simulink model "FinalV2"  (R2018b)
settings: Solver=FixedStepAuto  StartTime=0.0  StopTime=1  RelTol=1e-3
values from neighbouring files (symbols this model uses):
  Kdi = dlqr(Ad,Bd,Q,R)    [finalScript.m]    (also in finalScriptV2.m)
  n = 16.5    [DC_motor_geared_integral_discrete_sysid23.m]    (also in DC_motor_geared_lqr_discrete_sysid23.m; finalScript.m; finalScriptV2.m)
  Tsc = 1/20000    (= 5e-05)    [DC_motor_geared_integral_discrete_sysid23.m]    (also in DC_motor_geared_lqr_discrete_sysid23.m = 1e-05; finalScript.m; finalScriptV2.m = 0.001)
undefined symbols (not defined in the file or in its folder): DiscIntNeverNeededParam
libraries: dspswit3 x29, mbedblockslib x19, simulink x10, dspsigops x5, powerlib_meascontrol x4, dspstat3 x2, peGeneralControl x1
(part 1 of 2)
settings Model: Creator=Roberto  LastModifiedBy=Cas
settings SolverCC: AutoInsertRateTranBlk=on
settings OptimizationCC: DefaultParameterBehavior=Inlined  UseFloatMulNetSlope=on  UseSpecifiedMinMax=on  InlineInvariantSignals=on  PassReuseOutputArgsAs=Individual arguments  ZeroExternalMemoryAtStartup=off  ZeroInternalMemoryAtStartup=off  NoFixptDivByZeroProtection=on  EfficientFloat2IntCast=on  MaxStackSize=64  OptimizeBlockOrder=speed  DifferentSizesBufferReuse=on
settings DebuggingCC: ParameterTunabilityLossMsg=error
settings HardwareCC: ProdBitPerPointer=32  ProdBitPerSizeT=32  ProdBitPerPtrDiffT=32  ProdLargestAtomicInteger=Long  ProdLargestAtomicFloat=Double  ProdWordSize=32  ProdLongLongMode=on  ProdHWDeviceType=ARM Compatible->ARM Cortex
settings ModelReferenceCC: ModelReferenceMinAlgLoopOccurrences=on
settings SFSimCC: MATLABDynamicMemAlloc=off
settings RTWCC: SystemTargetFile=ert.tlc  HardwareBoard=STM32F746G-Discovery  TemplateMakefile=ert_default_tmf  GenerateReport=on  Toolchain=GNU Tools for ARM Embedded Processors  BuildConfiguration=Faster Runs  IncludeHyperlinkInReport=on  LaunchReport=on  GenerateTraceInfo=on  GenerateTraceReport=on  GenerateTraceReportSl=on  GenerateTraceReportSf=on  GenerateTraceReportEml=on
settings CodeAppCC: ForceParamTrailComments=on  IgnoreCustomStorageClasses=off  OperatorAnnotations=on  SimulinkDataObjDesc=on  SFDataObjDesc=on  InsertBlockDesc=on
settings ERTTargetCC: CombineSignalStateStructs=on  SuppressErrorStatus=on  SupportNonFinite=off

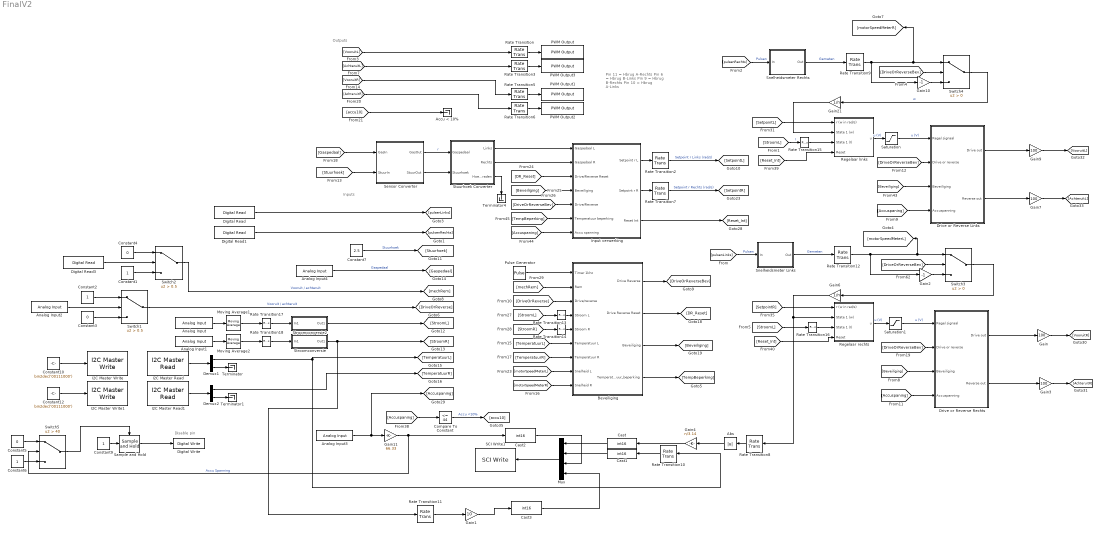
== system FinalV2 ==
  note: Disable pin
  note: Pin 11 = Hbrug A-Rechts
      | Pin 6   = Hbrug B-Links
      | Pin 9   = Hbrug B-Rechts
      | Pin 10 = Hbrug A-Links
  note: Inputs
  note: Outputs
  Abs : Abs
  Accu < 10% : Terminator
  Analog Input : mbedblockslib/Analog Input  Pin=A3  ReadResultsOnly=off  ConversionTriggerSource=Software  ExternalTriggerType=uint32( 0 )  OutputDataType=double  EnableConversionCompleteNotify=off  EnableOuputStatus=off  SampleTime=1/10000
      settings: SourceProductName=Simulink Coder Support Package for BBC microbit Board  SourceProductBaseCode=MICROBIT
  Analog Input1 : mbedblockslib/Analog Input  Pin=A2  ReadResultsOnly=off  ConversionTriggerSource=Software  ExternalTriggerType=uint32( 0 )  OutputDataType=double  EnableConversionCompleteNotify=off  EnableOuputStatus=off  SampleTime=1/10000
      settings: SourceProductName=Simulink Coder Support Package for BBC microbit Board  SourceProductBaseCode=MICROBIT
  Analog Input2 : mbedblockslib/Analog Input  Pin=A0  ReadResultsOnly=off  ConversionTriggerSource=Software  ExternalTriggerType=uint32( 0 )  OutputDataType=double  EnableConversionCompleteNotify=off  EnableOuputStatus=off  SampleTime=Tsc
      settings: SourceProductName=Simulink Coder Support Package for BBC microbit Board  SourceProductBaseCode=MICROBIT
  Analog Input3 : mbedblockslib/Analog Input  Pin=A1  ReadResultsOnly=off  ConversionTriggerSource=Software  ExternalTriggerType=uint32( 0 )  OutputDataType=double  EnableConversionCompleteNotify=off  EnableOuputStatus=off  SampleTime=1/20
      settings: SourceProductName=Simulink Coder Support Package for BBC microbit Board  SourceProductBaseCode=MICROBIT
  Analog Input4 : mbedblockslib/Analog Input  Pin=A4  ReadResultsOnly=off  ConversionTriggerSource=Software  ExternalTriggerType=uint32( 0 )  OutputDataType=double  EnableConversionCompleteNotify=off  EnableOuputStatus=off  SampleTime=Tsc
      settings: SourceProductName=Simulink Coder Support Package for BBC microbit Board  SourceProductBaseCode=MICROBIT
  Beveiliging : Subsystem
  Cast{,1..3} (4 alike) : DataTypeConversion  OutDataTypeStr=int16
  Compare To Constant : simulink/Logic and Bit Operations/Compare To Constant  relop=<=  const=44  OutDataTypeStr=boolean
  Constant1 : Constant  OutDataTypeStr=boolean  SampleTime=Tsc
  Constant10 : Constant  Value=bin2dec('00111000')  OutDataTypeStr=uint8  SampleTime=20
  Constant12 : Constant  Value=bin2dec('00111000')  OutDataTypeStr=uint8  SampleTime=20
  Constant2 : Constant  OutDataTypeStr=boolean  SampleTime=Tsc
  Constant3 : Constant  Value=0  OutDataTypeStr=boolean  SampleTime=Tsc
  Constant4 : Constant  Value=0  OutDataTypeStr=boolean  SampleTime=Tsc
  Constant5 : Constant  Value=0  OutDataTypeStr=boolean  SampleTime=1/20
  Constant6 : Constant  OutDataTypeStr=boolean  SampleTime=1/20
  Constant7 : Constant  Value=2.5  SampleTime=Tsc
  Constant9 : Constant  OutDataTypeStr=boolean  SampleTime=1/20
  Demux1 : Demux  Outputs=2
  Demux2 : Demux  Outputs=2
  Digital Read : mbedblockslib/Digital Read  Pin=4  Direction=input  SampleTime=1/200000
      settings: SourceProductName=Simulink Coder Support Package for BBC microbit Board  SourceProductBaseCode=MICROBIT
  Digital Read1 : mbedblockslib/Digital Read  Pin=5  Direction=input  SampleTime=1/200000
      settings: SourceProductName=Simulink Coder Support Package for BBC microbit Board  SourceProductBaseCode=MICROBIT
  Digital Read3 : mbedblockslib/Digital Read  Pin=2  Direction=input  SampleTime=Tsc
      settings: SourceProductName=Simulink Coder Support Package for BBC microbit Board  SourceProductBaseCode=MICROBIT
  Digital Write : mbedblockslib/Digital Write  Pin=7  Direction=output
      settings: SourceProductName=Simulink Coder Support Package for BBC microbit Board  SourceProductBaseCode=MICROBIT
  Drive or Reverse Links : Subsystem
  Drive or Reverse Rechts : Subsystem
  Gain{,3,7,9} (4 alike) : Gain  Gain=100
  Gain1 : Gain  Gain=10
  Gain10 : Gain  Gain=-1
  Gain11 : Gain  Gain=66.33
  Gain2 : Gain  Gain=-1
  Gain21 : Gain  Gain=1/n
  Gain4 : Gain  Gain=n/3.14
  Gain6 : Gain  Gain=1/n
  I2C Master Read : mbedblockslib/I2C Master Read  I2CModule=0  Mode=Master  SlaveAddress=bin2dec('1001001')  SlaveByteOrder=BigEndian  Direction=Receiver  RegisterAddressMode=on  RegisterAddress=uint8(0)  SlaveDataType=uint8  DataLength=2  NoAck=off  RepeatedStart=off  OutputStatus=off  SampleTime=1/1000
      settings: SourceProductName=Simulink Coder Support Package for BBC microbit Board  SourceProductBaseCode=MICROBIT
  I2C Master Read1 : mbedblockslib/I2C Master Read  I2CModule=0  Mode=Master  SlaveAddress=bin2dec('1001000')  SlaveByteOrder=BigEndian  Direction=Receiver  RegisterAddressMode=on  RegisterAddress=uint8(0)  SlaveDataType=uint8  DataLength=2  NoAck=off  RepeatedStart=off  OutputStatus=off  SampleTime=1/1000
      settings: SourceProductName=Simulink Coder Support Package for BBC microbit Board  SourceProductBaseCode=MICROBIT
  I2C Master Write : mbedblockslib/I2C Master Write  I2CModule=0  Mode=Master  SlaveAddress=bin2dec('1001001')  SlaveByteOrder=BigEndian  Direction=Transmitter  RegisterAddressMode=on  RegisterAddress=uint8(1)  SlaveDataType=uint8  DataLength=2  NoAck=off  RepeatedStart=off  OutputStatus=off
      settings: SourceProductName=Simulink Coder Support Package for BBC microbit Board  SourceProductBaseCode=MICROBIT
  I2C Master Write1 : mbedblockslib/I2C Master Write  I2CModule=0  Mode=Master  SlaveAddress=bin2dec('1001000')  SlaveByteOrder=BigEndian  Direction=Transmitter  RegisterAddressMode=on  RegisterAddress=uint8(1)  SlaveDataType=uint8  DataLength=2  NoAck=off  RepeatedStart=off  OutputStatus=off
      settings: SourceProductName=Simulink Coder Support Package for BBC microbit Board  SourceProductBaseCode=MICROBIT
  Input verwerking : Subsystem
  Moving Average1 : dspstat3/Moving Average  Method=Sliding window  ForgettingFactorPort=off  SpecifyWindowLength=on  WindowLength=20  ForgettingFactor=0.9  SimulateUsing=Code generation
  Moving Average2 : dspstat3/Moving Average  Method=Sliding window  ForgettingFactorPort=off  SpecifyWindowLength=on  WindowLength=20  ForgettingFactor=0.9  SimulateUsing=Code generation
  Mux : Mux
  PWM Output : mbedblockslib/PWM Output  Pin=10  EnableInputFrequency=off  InitialFrequency=20e3  InitialDutyCycle=0  NotificationType=None
      settings: SourceProductName=Simulink Coder Support Package for BBC microbit Board  SourceProductBaseCode=MICROBIT
  PWM Output1 : mbedblockslib/PWM Output  Pin=6  EnableInputFrequency=off  InitialFrequency=20e3  InitialDutyCycle=0  NotificationType=None
      settings: SourceProductName=Simulink Coder Support Package for BBC microbit Board  SourceProductBaseCode=MICROBIT
  PWM Output2 : mbedblockslib/PWM Output  Pin=9  EnableInputFrequency=off  InitialFrequency=20e3  InitialDutyCycle=0  NotificationType=None
      settings: SourceProductName=Simulink Coder Support Package for BBC microbit Board  SourceProductBaseCode=MICROBIT
  PWM Output3 : mbedblockslib/PWM Output  Pin=11  EnableInputFrequency=off  InitialFrequency=20e3  InitialDutyCycle=0  NotificationType=None
      settings: SourceProductName=Simulink Coder Support Package for BBC microbit Board  SourceProductBaseCode=MICROBIT
  Pulse Generator : DiscretePulseGenerator  SampleTime=1/1000
  Rate Transition{,3,5..6,8,10..11} (7 alike) : RateTransition  OutPortSampleTime=1/20
  Rate Transition{2,7,9,12,15..18} (8 alike) : RateTransition  OutPortSampleTime=Tsc
  Rate Transition13 : RateTransition  OutPortSampleTime=1/1000
  Rate Transition14 : RateTransition  OutPortSampleTime=1/1000
  Regelaar links : Subsystem
  Regelaar rechts : Subsystem
  SCI Write1 : mbedblockslib/SCI Write  SCIModule=0  Baudrate=uint32(9600)  Parity=None  StopBits=1  HardwareFlowControl=None  ByteOrder=LittleEndian  OutputStatus=off
      settings: SourceProductName=Simulink Coder Support Package for BBC microbit Board  SourceProductBaseCode=MICROBIT
  Sample and Hold : dspsigops/Sample and Hold  trig=Rising edge  initCond=0  latchinput=off
  Saturation : Saturate  UpperLimit=60  LowerLimit=-60  OutDataTypeStr=Inherit: Inherit via back propagation
  Saturation1 : Saturate  UpperLimit=60  LowerLimit=-60
  Sensor Converter : Subsystem
  Snelheidsmeter Links : Subsystem
  Snelheidsmeter Rechts : Subsystem
  Stroomconversie : Subsystem
  Stroomconversie2 : Subsystem
  Stuurhoek Converter : Subsystem
  Switch1 : Switch  Criteria=u2 > Threshold  Threshold=0.5
  Switch2 : Switch  Criteria=u2 > Threshold  Threshold=0.5
  Switch3 : Switch  Criteria=u2 > Threshold
  Switch4 : Switch  Criteria=u2 > Threshold
  Switch5 : Switch  Criteria=u2 > Threshold  Threshold=40
  Terminator : Terminator
  Terminator1 : Terminator
  Terminator4 : Terminator
  wires:
  [pulsenRechts] -> Snelheidsmeter Rechts/1(In)  "Pulsen"
  Beveiliging/1("Drive Reverse ") -> [DriveOrReverseBev]
  [Gaspedaal] -> Sensor Converter/1(GasIn)
  Stuurhoek Converter/1(Links) -> Input verwerking/1(Gaspedaal L)
  Input verwerking/1(Setpoint r L) -> Rate Transition2/1
  [Stuurhoek] -> Sensor Converter/2(StuurIn)
  Input verwerking/3(Reset Int) -> [Reset_Int]
  Sensor Converter/2(StuurOut) -> Stuurhoek Converter/2(Stuurhoek)
  [DriveOrReverse] -> Beveiliging/3(Drive/reverse)
  [TemperatuurL] -> Beveiliging/6(Temperatuur L)
  Beveiliging/3(Beveiliging) -> [Beveiliging]
  Input verwerking/2(Setpoint r R) -> Rate Transition7/1
  Beveiliging/2(Drive Reverse Reset) -> [DR_Reset]
  Stuurhoek Converter/2(Rechts) -> Input verwerking/2(Gaspedaal R)
  [mechRem] -> Beveiliging/2(Rem)
  [DR_Reset] -> Input verwerking/3(Drive/Reverse Reset)
  [Beveiliging] -> Input verwerking/4(Beveiliging)
  Pulse Generator/1 -> Beveiliging/1(Timer 1khz)
  [DriveOrReverseBev] -> Input verwerking/5(Drive/Reverse)
  Rate Transition7/1 -> [SetpointR]  "Setpoint r Rechts (rad/s)"
  Rate Transition2/1 -> [SetpointL]  "Setpoint r Links (rad/s)"
  [TemperatuurR] -> Beveiliging/7(Temperatuur R)
  Snelheidsmeter Links/1(Out) -> Rate Transition12/1  "Gemeten"
  [Reset_Int] -> Regelaar rechts/4(Reset)
  [pulsenLinks] -> Snelheidsmeter Links/1(In)  "Pulsen"
  [SetpointR] -> Regelaar rechts/1(r (w in rad/s))
  [Beveiliging] -> Drive or Reverse Rechts/3(Beveiliging)
  Drive or Reverse Rechts/1(Drive out) -> Gain/1
  [Accuspaning] -> Drive or Reverse Rechts/4(Accuspanning)
  [DriveOrReverseBev] -> Drive or Reverse Rechts/2(Drive or reverse)
  Drive or Reverse Rechts/2(Reverse out) -> Gain3/1
  Regelaar rechts/1(u) -> Saturation1/1  "u (V)"
  [Beveiliging] -> Drive or Reverse Links/3(Beveiliging)
  Drive or Reverse Links/1(Drive out) -> Gain9/1
  [Accuspaning] -> Drive or Reverse Links/4(Accuspanning)
  [DriveOrReverseBev] -> Drive or Reverse Links/2(Drive or reverse)
  Drive or Reverse Links/2(Reverse out) -> Gain7/1
  Regelaar links/1(u) -> Saturation/1  "u (V)"
  Switch1/1 -> [DriveOrReverse]  "Vooruit / achteruit"
  Constant7/1 -> [Stuurhoek]  "Stuurhoek"
  Beveiliging/4(Temperatuur_beperking) -> [TempBeperking]
  [Accuspaning] -> Input verwerking/7(Accu spanning)
  [TempBeperking] -> Input verwerking/6(Temperatuur beperking)
  [DriveOrReverseBev] -> Switch3/2
  Gain2/1 -> Switch3/3
  Gain10/1 -> Switch4/3
  [DriveOrReverseBev] -> Switch4/2
  Saturation/1 -> Drive or Reverse Links/1(Regel signaal)  "u (V)"
  Saturation1/1 -> Drive or Reverse Rechts/1(Regel signaal)  "u (V)"
  Compare To Constant/1 -> [accu10]  "Accu <10%"
  [Accuspaning] -> Compare To Constant/1
  Sensor Converter/1(GasOut) -> Stuurhoek Converter/1("Gaspedaal ")  "r"
  Stuurhoek Converter/3(Hoek in graden) -> Terminator4/1
  Gain/1 -> [VooruitR]
  Gain3/1 -> [AchteruitR]
  Gain7/1 -> [AchteruitL]
  Gain9/1 -> [VooruitL]
  [accu10] -> Accu < 10%/1
  [SetpointL] -> Regelaar links/1(r (w in rad/s))
  Switch4/1 -> Gain21/1  "w"
  [StroomL] -> Rate Transition15/1  "I"
  [Reset_Int] -> Regelaar links/4(Reset)
  Snelheidsmeter Rechts/1(Out) -> Rate Transition9/1  "Gemeten"
  [AchteruitR] -> Rate Transition6/1
  [VooruitR] -> Rate Transition5/1
  Rate Transition3/1 -> PWM Output3/1
  Rate Transition5/1 -> PWM Output1/1
  Rate Transition6/1 -> PWM Output2/1
  Rate Transition/1 -> PWM Output/1
  Digital Read/1 -> [pulsenLinks]
  Analog Input3/1 -> [Accuspaning], Gain11/1
  Analog Input4/1 -> [Gaspedaal]  "Gaspedaal"
  [StroomL] -> Rate Transition16/1
  Constant2/1 -> Switch1/1
  Constant3/1 -> Switch1/3
  Digital Read3/1 -> Switch2/2
  Constant1/1 -> Switch2/3
  Constant4/1 -> Switch2/1
  Switch2/1 -> [mechRem]  "Vooruit / achteruit"
  Analog Input2/1 -> Switch1/2
  I2C Master Read/1 -> Demux1/1
  Constant10/1 -> I2C Master Write/1
  Demux1/2 -> Terminator/1
  Stroomconversie2/1(Out1) -> [StroomL]
  [StroomL] -> Rate Transition13/1
  [StroomR] -> Rate Transition14/1
  Cast1/1 -> Mux/2
  Switch3/1 -> Gain6/1
  Abs/1 -> Gain4/1
  Mux/1 -> SCI Write1/1
  Rate Transition8/1 -> Abs/1
  Rate Transition10/1 -> Cast1/1
  Rate Transition11/1 -> Gain1/1
  Gain1/1 -> Cast3/1
  Gain11/1 -> Switch5/2, Cast2/1  "Accu Spanning"
  Constant6/1 -> Switch5/3
  Constant5/1 -> Switch5/1
  Switch5/1 -> Sample and Hold/Trigger
  Constant9/1 -> Sample and Hold/1
  Sample and Hold/1 -> Digital Write/1
  [VooruitL] -> Rate Transition/1
  [AchteruitL] -> Rate Transition3/1
  Gain4/1 -> Cast/1
  Gain6/1 -> Rate Transition8/1, Regelaar rechts/2(State 1 (w))
  Gain21/1 -> Regelaar links/2(State 1 (w))
  Constant12/1 -> I2C Master Write1/1
  I2C Master Read1/1 -> Demux2/1
  Demux2/2 -> Terminator1/1
  Demux2/1 -> [TemperatuurR]
  Rate Transition9/1 -> Gain10/1, [motorSpeedMeterR], Switch4/1
  Rate Transition12/1 -> Gain2/1, [motorSpeedMeterL], Switch3/1
  [motorSpeedMeterL] -> Beveiliging/8(Snelheid L)
  [motorSpeedMeterR] -> Beveiliging/9(Snelheid R)
  Rate Transition13/1 -> Beveiliging/4(Stroom L)
  Rate Transition14/1 -> Beveiliging/5(Stroom R)
  Rate Transition15/1 -> Regelaar links/3(State 1 (I))
  Rate Transition16/1 -> Regelaar rechts/3(State 1 (I))
  Analog Input/1 -> Moving Average1/1
  Analog Input1/1 -> Moving Average2/1
  Rate Transition17/1 -> Stroomconversie2/1(In1)
  Rate Transition18/1 -> Stroomconversie/1(In1)
  Stroomconversie/1(Out1) -> Rate Transition11/1, [StroomR]
  Moving Average1/1 -> Rate Transition17/1
  Moving Average2/1 -> Rate Transition18/1
  Demux1/1 -> Rate Transition10/1, [TemperatuurL]
  Cast/1 -> Mux/1
  Cast2/1 -> Mux/3
  Cast3/1 -> Mux/4
  Digital Read1/1 -> [pulsenRechts]

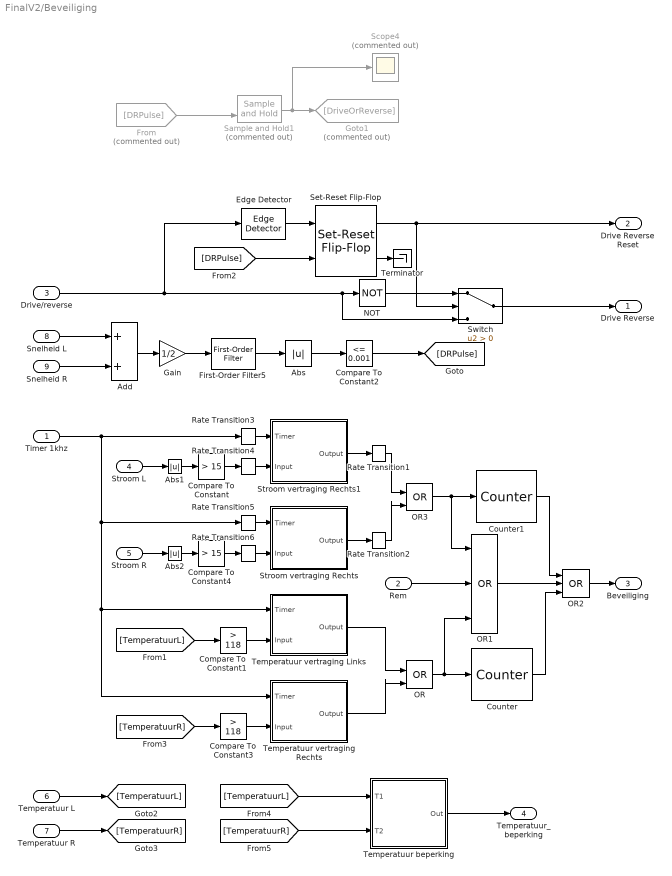
== system FinalV2/Beveiliging ==
  Timer 1khz : Inport
  Rem : Inport  Port=2
  Drive/reverse : Inport  Port=3
  Stroom L : Inport  Port=4
  Stroom R : Inport  Port=5
  Temperatuur L : Inport  Port=6
  Temperatuur R : Inport  Port=7
  Snelheid L : Inport  Port=8
  Snelheid R : Inport  Port=9
  Abs : Abs
  Abs1 : Abs
  Abs2 : Abs
  Add : Sum
  Compare To Constant : simulink/Logic and Bit Operations/Compare To Constant  relop=>  const=15  OutDataTypeStr=boolean
  Compare To Constant1 : simulink/Logic and Bit Operations/Compare To Constant  relop=>  const=118  OutDataTypeStr=boolean
  Compare To Constant2 : simulink/Logic and Bit Operations/Compare To Constant  relop=<=  const=0.001  OutDataTypeStr=boolean
  Compare To Constant3 : simulink/Logic and Bit Operations/Compare To Constant  relop=>  const=118  OutDataTypeStr=boolean
  Compare To Constant4 : simulink/Logic and Bit Operations/Compare To Constant  relop=>  const=15  OutDataTypeStr=boolean
  Counter : dspswit3/Counter  Direction=Up  CountEvent=Rising edge  CounterSize=32 bits  MaxCount=255  InitialCount=0  Output=Hit  HitValue=3  ResetInput=off  SamplesPerFrame=1  Ts=1  CntDtype=double  HitDtype=Logical
  Counter1 : dspswit3/Counter  Direction=Up  CountEvent=Rising edge  CounterSize=32 bits  MaxCount=255  InitialCount=0  Output=Hit  HitValue=2  ResetInput=off  SamplesPerFrame=1  Ts=1  CntDtype=double  HitDtype=Logical
  Edge Detector : powerlib_meascontrol/Logic/Edge Detector  model=Either  ic=0  Ts=-1
      settings: SourceProductName=Simscape Power Systems  SourceProductBaseCode=PS
  First-Order Filter5 : powerlib_meascontrol/Filters/First-Order Filter  FilterType=Lowpass  Tc=10e-3  Ts=Tsc  Initialize=on  Vac_Init=[0, 0, 50]  Vdc_Init=0  PlotResponse=off  FreqRange="[0,  200,  1]"
      settings: SourceProductName=Simscape Power Systems
  From : From  Commented=on  GotoTag=DRPulse
  Gain : Gain  Gain=1/2
  Goto1 : Goto  Commented=on  GotoTag=DriveOrReverse
  NOT : Logic  Operator=NOT  IconShape=distinctive  AllPortsSameDT=off  OutDataTypeStr=boolean
  OR : Logic  Operator=OR  IconShape=distinctive  AllPortsSameDT=off  OutDataTypeStr=boolean
  OR1 : Logic  Operator=OR  Inputs=3  IconShape=distinctive  AllPortsSameDT=off  OutDataTypeStr=boolean
  OR2 : Logic  Operator=OR  Inputs=3  IconShape=distinctive  AllPortsSameDT=off  OutDataTypeStr=boolean
  OR3 : Logic  Operator=OR  IconShape=distinctive  AllPortsSameDT=off  OutDataTypeStr=boolean
  Rate Transition{1..6} (6 alike) : RateTransition
  Sample and Hold1 : powerlib_meascontrol/Additional Components/Sample and Hold  Commented=on  ic=0  Ts=0
      settings: SourceProductName=Simscape Power Systems  SourceProductBaseCode=PS
  Scope4 : Scope  Commented=on
  Set-Reset Flip-Flop : peGeneralControl/Set-Reset Flip-Flop  LabelModeActiveChoice=Discrete  UndefState=Set  Q0=0  Ts=-1
  Stroom vertraging Rechts : Subsystem
  Stroom vertraging Rechts1 : Subsystem
  Switch : Switch  Criteria=u2 > Threshold
  Temperatuur beperking : Subsystem
  Temperatuur vertraging Links : Subsystem
  "Temperatuur vertraging Rechts " : Subsystem
  Terminator : Terminator
  "Drive Reverse " : Outport
  Drive Reverse Reset : Outport  Port=2
  Beveiliging : Outport  Port=3
  Temperatuur_beperking : Outport  Port=4
  wires:
  Compare To Constant1/1 -> Temperatuur vertraging Links/2(Input)
  Edge Detector/1 -> Set-Reset Flip-Flop/1
  Set-Reset Flip-Flop/1 -> Switch/2, Drive Reverse Reset/1
  Sample and Hold1/1 -> Scope4/1, Goto1/1
  Abs/1 -> Compare To Constant2/1
  Compare To Constant2/1 -> [DRPulse]
  Drive/reverse/1 -> Edge Detector/1, Switch/3, NOT/1
  From/1 -> Sample and Hold1/2
  Snelheid L/1 -> Add/1
  Snelheid R/1 -> Add/2
  Add/1 -> Gain/1
  Compare To Constant3/1 -> "Temperatuur vertraging Rechts "/2(Input)
  Timer 1khz/1 -> Rate Transition3/1, Rate Transition5/1, Temperatuur vertraging Links/1(Timer), "Temperatuur vertraging Rechts "/1(Timer)
  Rem/1 -> OR1/2
  Switch/1 -> "Drive Reverse "/1
  NOT/1 -> Switch/1
  OR/1 -> OR1/3, Counter/1
  Temperatuur vertraging Links/1(Output) -> OR/1
  "Temperatuur vertraging Rechts "/1(Output) -> OR/2
  OR2/1 -> Beveiliging/1
  Counter/1 -> OR2/3
  OR1/1 -> OR2/2
  Set-Reset Flip-Flop/2 -> Terminator/1
  Temperatuur L/1 -> [TemperatuurL]
  Temperatuur R/1 -> [TemperatuurR]
  [TemperatuurL] -> Compare To Constant1/1
  [TemperatuurR] -> Compare To Constant3/1
  [TemperatuurL] -> Temperatuur beperking/1(T1)
  [TemperatuurR] -> Temperatuur beperking/2(T2)
  Temperatuur beperking/1(Out) -> Temperatuur_beperking/1
  Stroom vertraging Rechts1/1(Output) -> Rate Transition1/1
  Stroom vertraging Rechts/1(Output) -> Rate Transition2/1
  OR3/1 -> Counter1/1, OR1/1
  Counter1/1 -> OR2/1
  Rate Transition6/1 -> Stroom vertraging Rechts/2(Input)
  Rate Transition5/1 -> Stroom vertraging Rechts/1(Timer)
  Rate Transition4/1 -> Stroom vertraging Rechts1/2(Input)
  Rate Transition3/1 -> Stroom vertraging Rechts1/1(Timer)
  Rate Transition2/1 -> OR3/2
  Rate Transition1/1 -> OR3/1
  Compare To Constant/1 -> Rate Transition4/1
  Compare To Constant4/1 -> Rate Transition6/1
  Stroom L/1 -> Abs1/1
  Stroom R/1 -> Abs2/1
  Abs1/1 -> Compare To Constant/1
  Abs2/1 -> Compare To Constant4/1
  First-Order Filter5/1 -> Abs/1
  Gain/1 -> First-Order Filter5/1
  [DRPulse] -> Set-Reset Flip-Flop/2

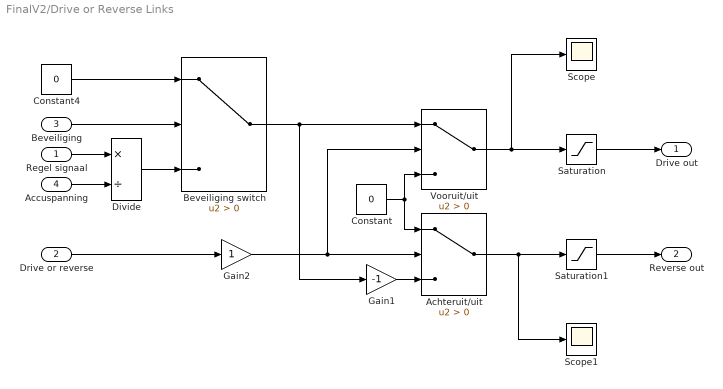
== system FinalV2/Drive or Reverse Links ==
  Regel signaal : Inport
  Drive or reverse : Inport  Port=2
  Beveiliging : Inport  Port=3
  Accuspanning : Inport  Port=4
  Achteruit/uit : Switch  Criteria=u2 > Threshold
  Beveiliging switch : Switch  Criteria=u2 > Threshold
  Constant : Constant  Value=0  SampleTime=Tsc
  Constant4 : Constant  Value=0  SampleTime=Tsc
  Divide : Product  Inputs=*/
  Gain1 : Gain  Gain=-1
  Gain2 : Gain
  Saturation : Saturate  UpperLimit=1  LowerLimit=0
  Saturation1 : Saturate  UpperLimit=1  LowerLimit=0
  Scope : Scope
  Scope1 : Scope
  Vooruit/uit : Switch  Criteria=u2 > Threshold
  Drive out : Outport
  Reverse out : Outport  Port=2
  wires:
  Gain1/1 -> Achteruit/uit/3
  Constant4/1 -> Beveiliging switch/1
  Constant/1 -> Achteruit/uit/1, Vooruit/uit/3
  Beveiliging switch/1 -> Gain1/1, Vooruit/uit/1
  Beveiliging/1 -> Beveiliging switch/2
  Achteruit/uit/1 -> Saturation1/1, Scope1/1
  Gain2/1 -> Vooruit/uit/2, Achteruit/uit/2
  Drive or reverse/1 -> Gain2/1
  Vooruit/uit/1 -> Saturation/1, Scope/1
  Accuspanning/1 -> Divide/2
  Divide/1 -> Beveiliging switch/3
  Regel signaal/1 -> Divide/1
  Saturation/1 -> Drive out/1
  Saturation1/1 -> Reverse out/1

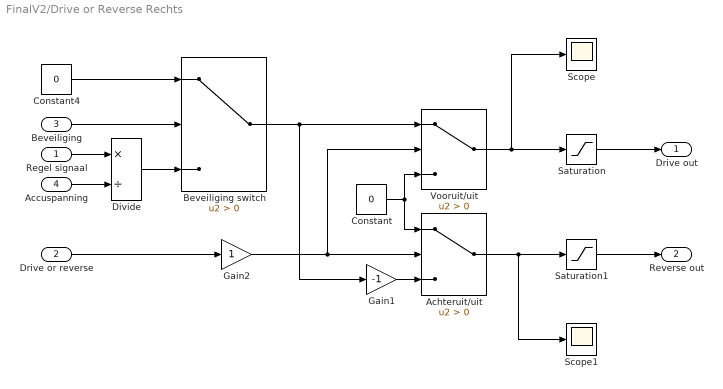
== system FinalV2/Drive or Reverse Rechts ==
  Regel signaal : Inport
  Drive or reverse : Inport  Port=2
  Beveiliging : Inport  Port=3
  Accuspanning : Inport  Port=4
  Achteruit/uit : Switch  Criteria=u2 > Threshold
  Beveiliging switch : Switch  Criteria=u2 > Threshold
  Constant : Constant  Value=0
  Constant4 : Constant  Value=0
  Divide : Product  Inputs=*/
  Gain1 : Gain  Gain=-1
  Gain2 : Gain
  Saturation : Saturate  UpperLimit=1  LowerLimit=0
  Saturation1 : Saturate  UpperLimit=1  LowerLimit=0
  Scope : Scope
  Scope1 : Scope
  Vooruit/uit : Switch  Criteria=u2 > Threshold
  Drive out : Outport
  Reverse out : Outport  Port=2
  wires:
  Gain1/1 -> Achteruit/uit/3
  Constant4/1 -> Beveiliging switch/1
  Constant/1 -> Achteruit/uit/1, Vooruit/uit/3
  Beveiliging switch/1 -> Gain1/1, Vooruit/uit/1
  Beveiliging/1 -> Beveiliging switch/2
  Achteruit/uit/1 -> Saturation1/1, Scope1/1
  Gain2/1 -> Vooruit/uit/2, Achteruit/uit/2
  Drive or reverse/1 -> Gain2/1
  Vooruit/uit/1 -> Saturation/1, Scope/1
  Accuspanning/1 -> Divide/2
  Divide/1 -> Beveiliging switch/3
  Regel signaal/1 -> Divide/1
  Saturation/1 -> Drive out/1
  Saturation1/1 -> Reverse out/1

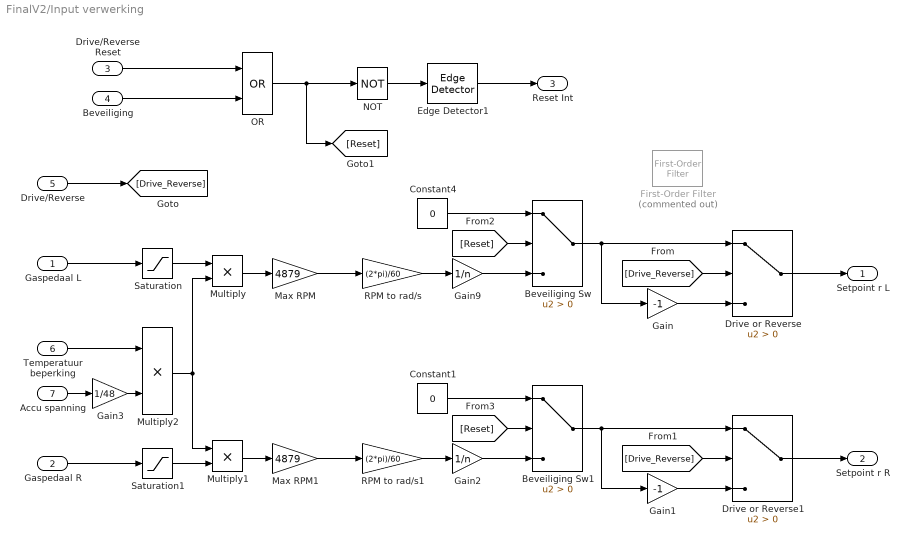
== system FinalV2/Input verwerking ==
  Gaspedaal L : Inport
  Gaspedaal R : Inport  Port=2
  Drive/Reverse Reset : Inport  Port=3
  Beveiliging : Inport  Port=4
  Drive/Reverse : Inport  Port=5
  Temperatuur beperking : Inport  Port=6
  Accu spanning : Inport  Port=7
  Beveiliging Sw : Switch  Criteria=u2 > Threshold
  Beveiliging Sw1 : Switch  Criteria=u2 > Threshold
  Constant1 : Constant  Value=0
  Constant4 : Constant  Value=0
  Drive or Reverse : Switch  Criteria=u2 > Threshold
  Drive or Reverse1 : Switch  Criteria=u2 > Threshold
  Edge Detector1 : dspswit3/Edge Detector  InputProcessing=Columns as channels (frame based)
      settings: SourceProductName=DSP System Toolbox  SourceProductBaseCode=DS
  First-Order Filter : powerlib_meascontrol/Filters/First-Order Filter  Commented=on  FilterType=Lowpass  Tc=10e-2  Ts=0  Initialize=on  Vac_Init=[0, 0, 60]  Vdc_Init=0  PlotResponse=off  FreqRange="[0,  200,  1]"
      settings: SourceProductName=Simscape Power Systems
  Gain : Gain  Gain=-1
  Gain1 : Gain  Gain=-1
  Gain2 : Gain  Gain=1/n
  Gain3 : Gain  Gain=1/48
  Gain9 : Gain  Gain=1/n
  Max RPM : Gain  Gain=4879
  Max RPM1 : Gain  Gain=4879
  Multiply : Product
  Multiply1 : Product
  Multiply2 : Product
  NOT : Logic  Operator=NOT  IconShape=distinctive  AllPortsSameDT=off  OutDataTypeStr=boolean
  OR : Logic  Operator=OR  IconShape=distinctive  AllPortsSameDT=off  OutDataTypeStr=boolean
  RPM to rad/s : Gain  Gain=(2*pi)/60
  RPM to rad/s1 : Gain  Gain=(2*pi)/60
  Saturation : Saturate  UpperLimit=1  LowerLimit=0
  Saturation1 : Saturate  UpperLimit=1  LowerLimit=0
  Setpoint r L : Outport
  Setpoint r R : Outport  Port=2
  Reset Int : Outport  Port=3
  wires:
  Constant4/1 -> Beveiliging Sw/1
  Max RPM/1 -> RPM to rad/s/1
  RPM to rad/s/1 -> Gain9/1
  Gaspedaal L/1 -> Saturation/1
  OR/1 -> [Reset], NOT/1
  Gain9/1 -> Beveiliging Sw/3
  Beveiliging Sw/1 -> Gain/1, Drive or Reverse/1
  Gain/1 -> Drive or Reverse/3
  [Drive_Reverse] -> Drive or Reverse/2
  Drive or Reverse/1 -> Setpoint r L/1
  Edge Detector1/1 -> Reset Int/1
  NOT/1 -> Edge Detector1/1
  Beveiliging/1 -> OR/2
  Drive/Reverse Reset/1 -> OR/1
  Max RPM1/1 -> RPM to rad/s1/1
  RPM to rad/s1/1 -> Gain2/1
  Drive or Reverse1/1 -> Setpoint r R/1
  Gaspedaal R/1 -> Saturation1/1
  Gain1/1 -> Drive or Reverse1/3
  Beveiliging Sw1/1 -> Gain1/1, Drive or Reverse1/1
  Constant1/1 -> Beveiliging Sw1/1
  [Drive_Reverse] -> Drive or Reverse1/2
  Gain2/1 -> Beveiliging Sw1/3
  Drive/Reverse/1 -> [Drive_Reverse]
  [Reset] -> Beveiliging Sw/2
  [Reset] -> Beveiliging Sw1/2
  Multiply/1 -> Max RPM/1
  Multiply1/1 -> Max RPM1/1
  Saturation1/1 -> Multiply1/2
  Saturation/1 -> Multiply/1
  Multiply2/1 -> Multiply/2, Multiply1/1
  Temperatuur beperking/1 -> Multiply2/1
  Accu spanning/1 -> Gain3/1
  Gain3/1 -> Multiply2/2

== system FinalV2/Regelaar links ==
  r (w in rad/s) : Inport
  State 1 (w) : Inport  Port=2
  State 1 (I) : Inport  Port=3
  Reset : Inport  Port=4
  Discrete-Time Integrator2 : DiscreteIntegrator  gainval=1  ExternalReset=rising  SampleTime=Tsc  ICPrevOutput=DiscIntNeverNeededParam  ICPrevScaledInput=DiscIntNeverNeededParam
  Gain1 : Gain  Gain=Kdi(1:2)  Multiplication=Matrix(K*u)
  Gain4 : Gain  Gain=Kdi(3)
  Mux : Mux  Inputs=2
  Sum1 : Sum  Inputs=|+-
  Sum4 : Sum  Inputs=|+-
  u : Outport
  wires:
  r (w in rad/s)/1 -> Sum1/1
  State 1 (I)/1 -> Mux/2
  Mux/1 -> Gain1/1
  Gain1/1 -> Sum4/2
  Gain4/1 -> Sum4/1
  Sum4/1 -> u/1
  State 1 (w)/1 -> Mux/1, Sum1/2
  Sum1/1 -> Discrete-Time Integrator2/1
  Discrete-Time Integrator2/1 -> Gain4/1
  Reset/1 -> Discrete-Time Integrator2/2

== system FinalV2/Regelaar rechts ==
  r (w in rad/s) : Inport
  State 1 (w) : Inport  Port=2
  State 1 (I) : Inport  Port=3
  Reset : Inport  Port=4
  Discrete-Time Integrator2 : DiscreteIntegrator  gainval=1  ExternalReset=rising  SampleTime=Tsc  ICPrevOutput=DiscIntNeverNeededParam  ICPrevScaledInput=DiscIntNeverNeededParam
  Gain1 : Gain  Gain=Kdi(1:2)  Multiplication=Matrix(K*u)
  Gain4 : Gain  Gain=Kdi(3)
  Mux : Mux  Inputs=2
  Sum1 : Sum  Inputs=|+-
  Sum4 : Sum  Inputs=|+-
  u : Outport
  wires:
  r (w in rad/s)/1 -> Sum1/1
  State 1 (I)/1 -> Mux/2
  Mux/1 -> Gain1/1
  Gain1/1 -> Sum4/2
  Gain4/1 -> Sum4/1
  Sum4/1 -> u/1
  State 1 (w)/1 -> Mux/1, Sum1/2
  Sum1/1 -> Discrete-Time Integrator2/1
  Discrete-Time Integrator2/1 -> Gain4/1
  Reset/1 -> Discrete-Time Integrator2/2

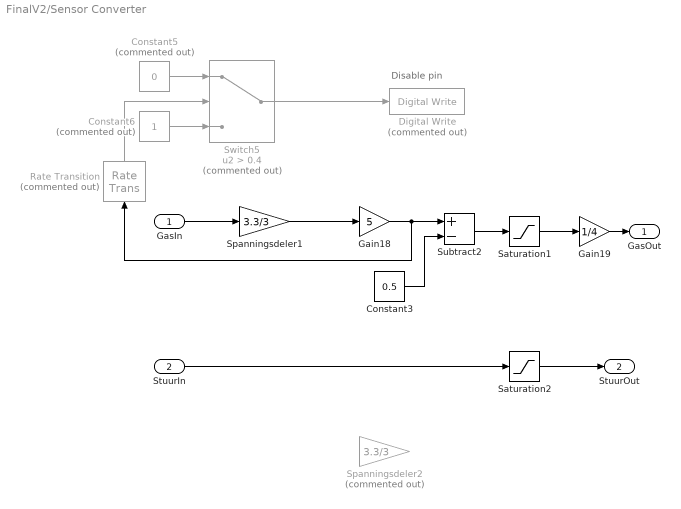
== system FinalV2/Sensor Converter ==
  note: Disable pin
  GasIn : Inport
  StuurIn : Inport  Port=2
  Constant3 : Constant  Value=0.5  SampleTime=1/1000
  Constant5 : Constant  Commented=on  Value=0  OutDataTypeStr=boolean  SampleTime=1/20
  Constant6 : Constant  Commented=on  OutDataTypeStr=boolean  SampleTime=1/20
  Digital Write : mbedblockslib/Digital Write  Commented=on  Pin=7  Direction=output
      settings: SourceProductName=Simulink Coder Support Package for BBC microbit Board  SourceProductBaseCode=MICROBIT
  Gain18 : Gain  Gain=5
  Gain19 : Gain  Gain=1/4
  Rate Transition : RateTransition  Commented=on  OutPortSampleTime=1/20
  Saturation1 : Saturate  UpperLimit=4  LowerLimit=0
  Saturation2 : Saturate  UpperLimit=1  LowerLimit=0
  Spanningsdeler1 : Gain  Gain=3.3/3
  Spanningsdeler2 : Gain  Commented=on  Gain=3.3/3
  Subtract2 : Sum  Inputs=+-
  Switch5 : Switch  Commented=on  Criteria=u2 > Threshold  Threshold=0.4
  GasOut : Outport
  StuurOut : Outport  Port=2
  wires:
  Constant3/1 -> Subtract2/2
  Saturation1/1 -> Gain19/1
  GasIn/1 -> Spanningsdeler1/1
  Gain18/1 -> Rate Transition/1, Subtract2/1
  Gain19/1 -> GasOut/1
  Subtract2/1 -> Saturation1/1
  Saturation2/1 -> StuurOut/1
  StuurIn/1 -> Saturation2/1
  Spanningsdeler1/1 -> Gain18/1
  Constant5/1 -> Switch5/1
  Constant6/1 -> Switch5/3
  Switch5/1 -> Digital Write/1
  Rate Transition/1 -> Switch5/2

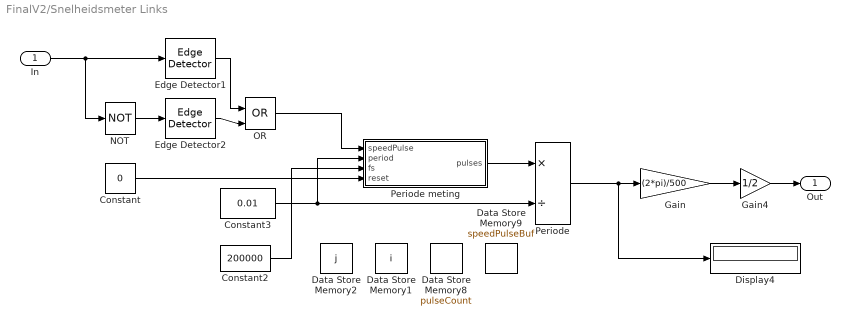
== system FinalV2/Snelheidsmeter Links ==
  In : Inport
  Constant : Constant  Value=0
  Constant2 : Constant  Value=200000
  Constant3 : Constant  Value=0.01
  Data Store Memory1 : DataStoreMemory  DataStoreName=i  ReadBeforeWriteMsg=warning  WriteAfterWriteMsg=warning  WriteAfterReadMsg=warning  InitialValue=1  ShowAdditionalParam=off  OutDataTypeStr=uint32
  Data Store Memory2 : DataStoreMemory  DataStoreName=j  ReadBeforeWriteMsg=warning  WriteAfterWriteMsg=warning  WriteAfterReadMsg=warning  InitialValue=2  ShowAdditionalParam=off  OutDataTypeStr=uint32
  Data Store Memory8 : DataStoreMemory  DataStoreName=pulseCount  ReadBeforeWriteMsg=warning  WriteAfterWriteMsg=warning  WriteAfterReadMsg=warning  ShowAdditionalParam=off  OutDataTypeStr=uint32
  Data Store Memory9 : DataStoreMemory  DataStoreName=speedPulseBuf  ReadBeforeWriteMsg=warning  WriteAfterWriteMsg=warning  WriteAfterReadMsg=warning  ShowAdditionalParam=off  OutDataTypeStr=uint8  Dimensions=10001
  Display4 : Display
  Edge Detector1 : dspswit3/Edge Detector  InputProcessing=Columns as channels (frame based)
      settings: SourceProductName=DSP System Toolbox  SourceProductBaseCode=DS
  Edge Detector2 : dspswit3/Edge Detector  InputProcessing=Columns as channels (frame based)
      settings: SourceProductName=DSP System Toolbox  SourceProductBaseCode=DS
  Gain : Gain  Gain=(2*pi)/500
  Gain4 : Gain  Gain=1/2
  NOT : Logic  Operator=NOT  IconShape=distinctive  AllPortsSameDT=off  OutDataTypeStr=boolean
  OR : Logic  Operator=OR  IconShape=distinctive  AllPortsSameDT=off  OutDataTypeStr=boolean
  Periode : Product  Inputs=*/
  Periode meting : MATLAB Function  TreatAsAtomicUnit=on
  Out : Outport
  wires:
  Constant3/1 -> Periode/2, Periode meting/2(period)
  Periode/1 -> Gain/1, Display4/1
  Constant2/1 -> Periode meting/3(fs)
  Periode meting/1(pulses) -> Periode/1
  In/1 -> NOT/1, Edge Detector1/1
  Gain/1 -> Gain4/1
  Constant/1 -> Periode meting/4(reset)
  OR/1 -> Periode meting/1(speedPulse)
  Edge Detector1/1 -> OR/1
  Edge Detector2/1 -> OR/2
  NOT/1 -> Edge Detector2/1
  Gain4/1 -> Out/1

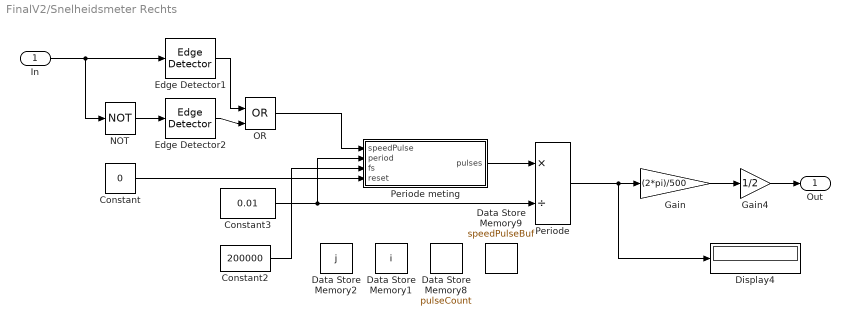
== system FinalV2/Snelheidsmeter Rechts ==
  In : Inport
  Constant : Constant  Value=0
  Constant2 : Constant  Value=200000
  Constant3 : Constant  Value=0.01
  Data Store Memory1 : DataStoreMemory  DataStoreName=i  ReadBeforeWriteMsg=warning  WriteAfterWriteMsg=warning  WriteAfterReadMsg=warning  InitialValue=1  ShowAdditionalParam=off  OutDataTypeStr=uint32
  Data Store Memory2 : DataStoreMemory  DataStoreName=j  ReadBeforeWriteMsg=warning  WriteAfterWriteMsg=warning  WriteAfterReadMsg=warning  InitialValue=2  ShowAdditionalParam=off  OutDataTypeStr=uint32
  Data Store Memory8 : DataStoreMemory  DataStoreName=pulseCount  ReadBeforeWriteMsg=warning  WriteAfterWriteMsg=warning  WriteAfterReadMsg=warning  ShowAdditionalParam=off  OutDataTypeStr=uint32
  Data Store Memory9 : DataStoreMemory  DataStoreName=speedPulseBuf  ReadBeforeWriteMsg=warning  WriteAfterWriteMsg=warning  WriteAfterReadMsg=warning  ShowAdditionalParam=off  OutDataTypeStr=uint8  Dimensions=10001
  Display4 : Display
  Edge Detector1 : dspswit3/Edge Detector  InputProcessing=Columns as channels (frame based)
      settings: SourceProductName=DSP System Toolbox  SourceProductBaseCode=DS
  Edge Detector2 : dspswit3/Edge Detector  InputProcessing=Columns as channels (frame based)
      settings: SourceProductName=DSP System Toolbox  SourceProductBaseCode=DS
  Gain : Gain  Gain=(2*pi)/500
  Gain4 : Gain  Gain=1/2
  NOT : Logic  Operator=NOT  IconShape=distinctive  AllPortsSameDT=off  OutDataTypeStr=boolean
  OR : Logic  Operator=OR  IconShape=distinctive  AllPortsSameDT=off  OutDataTypeStr=boolean
  Periode : Product  Inputs=*/
  Periode meting : MATLAB Function  TreatAsAtomicUnit=on
  Out : Outport
  wires:
  Constant3/1 -> Periode/2, Periode meting/2(period)
  Periode/1 -> Gain/1, Display4/1
  Constant2/1 -> Periode meting/3(fs)
  Periode meting/1(pulses) -> Periode/1
  In/1 -> NOT/1, Edge Detector1/1
  Gain/1 -> Gain4/1
  Constant/1 -> Periode meting/4(reset)
  OR/1 -> Periode meting/1(speedPulse)
  Edge Detector1/1 -> OR/1
  Edge Detector2/1 -> OR/2
  NOT/1 -> Edge Detector2/1
  Gain4/1 -> Out/1

== system FinalV2/Stroomconversie ==
  In1 : Inport
  Constant2 : Constant  Value=1.647  SampleTime=Tsc
  Gain : Gain  Gain=3.3
  Gain11 : Gain  Gain=1/0.055
  Subtract : Sum  Inputs=+-
  Out1 : Outport
  wires:
  In1/1 -> Gain/1
  Constant2/1 -> Subtract/2
  Subtract/1 -> Gain11/1
  Gain/1 -> Subtract/1
  Gain11/1 -> Out1/1

== system FinalV2/Stroomconversie2 ==
  note: Resolutie
  note: Offset weghalen
  In1 : Inport
  Constant2 : Constant  Value=1.647  SampleTime=Tsc
  Gain : Gain  Gain=3.3
  Gain11 : Gain  Gain=1/0.055
  Subtract : Sum  Inputs=+-
  Out1 : Outport
  wires:
  In1/1 -> Gain/1
  Gain11/1 -> Out1/1  "Stroom Links"
  Constant2/1 -> Subtract/2
  Subtract/1 -> Gain11/1
  Gain/1 -> Subtract/1

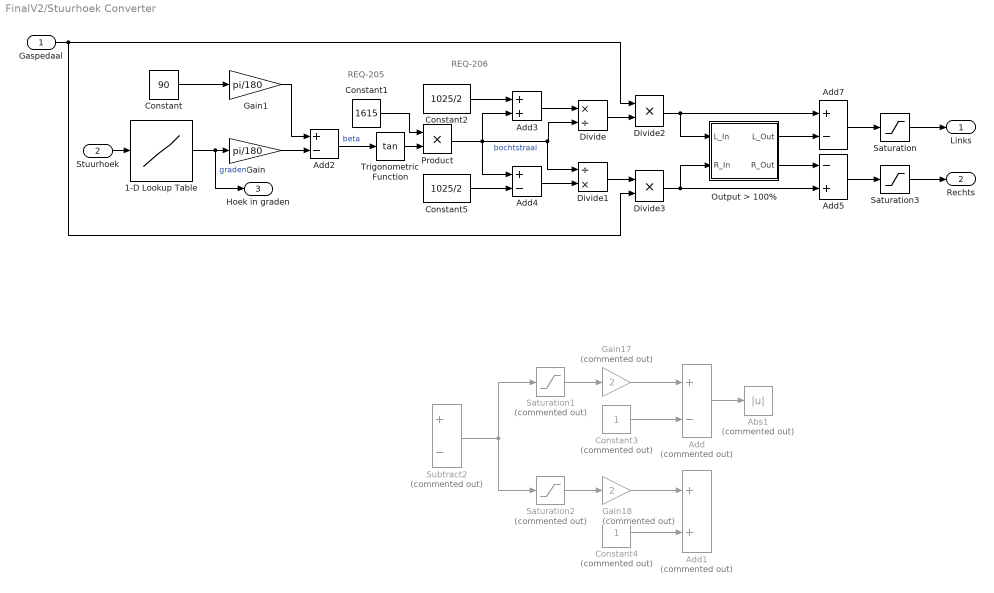
== system FinalV2/Stuurhoek Converter ==
  note: REQ-205
  note: REQ-206
  "Gaspedaal " : Inport
  Stuurhoek : Inport  Port=2
  1-D Lookup Table : Lookup_n-D  NumberOfTableDimensions=1  BreakpointsForDimension1=[0 0.5 1]  Table=[-30 0 30]  InternalRulePriority=Speed  RndMeth=Simplest  InputSameDT=on
  Abs1 : Abs  Commented=on
  Add : Sum  Commented=on  Inputs=+-
  Add1 : Sum  Commented=on
  Add2 : Sum  Inputs=+-
  Add3 : Sum
  Add4 : Sum  Inputs=+-
  Add5 : Sum  Inputs=-+
  Add7 : Sum  Inputs=+-
  Constant : Constant  Value=90
  Constant1 : Constant  Value=1615
  Constant2 : Constant  Value=1025/2
  Constant3 : Constant  Commented=on
  Constant4 : Constant  Commented=on
  Constant5 : Constant  Value=1025/2
  Divide : Product  Inputs=*/
  Divide1 : Product  Inputs=/*
  Divide2 : Product  Inputs=**
  Divide3 : Product  Inputs=**
  Gain : Gain  Gain=pi/180
  Gain1 : Gain  Gain=pi/180
  Gain17 : Gain  Commented=on  Gain=2
  Gain18 : Gain  Commented=on  Gain=2
  Output > 100% : Subsystem
  Product : Product
  Saturation : Saturate  UpperLimit=1  LowerLimit=0
  Saturation1 : Saturate  Commented=on  LowerLimit=0
  Saturation2 : Saturate  Commented=on  UpperLimit=0
  Saturation3 : Saturate  UpperLimit=1  LowerLimit=0
  Subtract2 : Sum  Commented=on  Inputs=+-
  Trigonometric Function : Trigonometry  Operator=tan
  Links : Outport
  Rechts : Outport  Port=2
  Hoek in graden : Outport  Port=3
  wires:
  Saturation1/1 -> Gain17/1
  Subtract2/1 -> Saturation2/1, Saturation1/1
  Gain18/1 -> Add1/1
  Add/1 -> Abs1/1
  Saturation2/1 -> Gain18/1
  Gain17/1 -> Add/1
  Constant4/1 -> Add1/2
  Constant3/1 -> Add/2
  1-D Lookup Table/1 -> Hoek in graden/1, Gain/1  "graden"
  Constant/1 -> Gain1/1
  Add2/1 -> Trigonometric Function/1  "beta"
  Constant1/1 -> Product/1
  Trigonometric Function/1 -> Product/2
  Product/1 -> Divide1/1, Divide/2, Add4/1, Add3/2  "bochtstraal"
  Constant2/1 -> Add3/1
  Add3/1 -> Divide/1
  Constant5/1 -> Add4/2
  Add4/1 -> Divide1/2
  Divide1/1 -> Divide3/1
  Divide/1 -> Divide2/2
  "Gaspedaal "/1 -> Divide2/1, Divide3/2
  Divide2/1 -> Add7/1, Output > 100%/1(L_In)
  Divide3/1 -> Output > 100%/2(R_In), Add5/2
  Stuurhoek/1 -> 1-D Lookup Table/1
  Gain/1 -> Add2/2
  Gain1/1 -> Add2/1
  Add7/1 -> Saturation/1
  Add5/1 -> Saturation3/1
  Output > 100%/1(L_Out) -> Add7/2
  Output > 100%/2(R_Out) -> Add5/1
  Saturation/1 -> Links/1
  Saturation3/1 -> Rechts/1

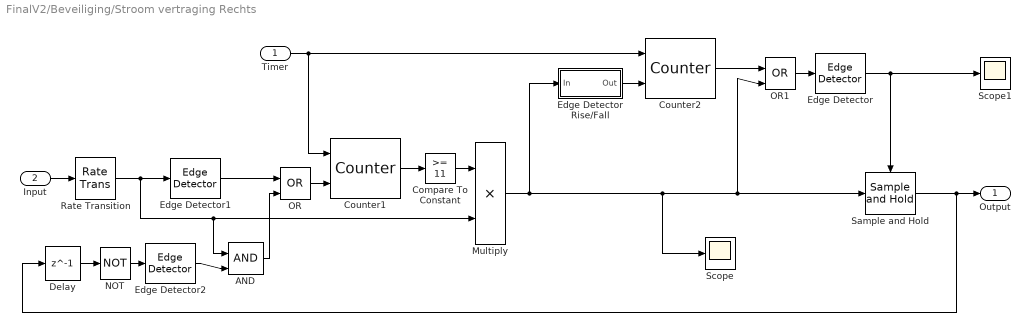
== system FinalV2/Beveiliging/Stroom vertraging Rechts ==
  Timer : Inport
  Input : Inport  Port=2
  AND : Logic  IconShape=distinctive  AllPortsSameDT=off  OutDataTypeStr=boolean
  Compare To Constant : simulink/Logic and Bit Operations/Compare To Constant  relop=>=  const=11  OutDataTypeStr=boolean
  Counter1 : dspswit3/Counter  Direction=Up  CountEvent=Rising edge  CounterSize=32 bits  MaxCount=20  InitialCount=0  Output=Count  HitValue=20  ResetInput=on  SamplesPerFrame=1  Ts=1  CntDtype=double  HitDtype=Logical
  Counter2 : dspswit3/Counter  Direction=Up  CountEvent=Rising edge  CounterSize=User defined  MaxCount=201  InitialCount=0  Output=Hit  HitValue=201  ResetInput=on  SamplesPerFrame=1  Ts=1  CntDtype=double  HitDtype=Logical
  Delay : Delay  DelayLength=1
  Edge Detector : dspswit3/Edge Detector  InputProcessing=Columns as channels (frame based)
      settings: SourceProductName=DSP System Toolbox  SourceProductBaseCode=DS
  Edge Detector1 : dspswit3/Edge Detector  InputProcessing=Columns as channels (frame based)
      settings: SourceProductName=DSP System Toolbox  SourceProductBaseCode=DS
  Edge Detector2 : dspswit3/Edge Detector  InputProcessing=Columns as channels (frame based)
      settings: SourceProductName=DSP System Toolbox  SourceProductBaseCode=DS
  Edge Detector Rise/Fall : Subsystem
  Multiply : Product
  NOT : Logic  Operator=NOT  IconShape=distinctive  AllPortsSameDT=off  OutDataTypeStr=boolean
  OR : Logic  Operator=OR  IconShape=distinctive  AllPortsSameDT=off  OutDataTypeStr=boolean
  OR1 : Logic  Operator=OR  IconShape=distinctive  AllPortsSameDT=off  OutDataTypeStr=boolean
  Rate Transition : RateTransition  OutPortSampleTime=1/1000
  Sample and Hold : dspsigops/Sample and Hold  trig=Rising edge  initCond=0  latchinput=off
  Scope : Scope
  Scope1 : Scope
  Output : Outport
  wires:
  Timer/1 -> Counter2/1, Counter1/1
  Sample and Hold/1 -> Output/1, Delay/1
  OR1/1 -> Edge Detector/1
  Edge Detector/1 -> Scope1/1, Sample and Hold/Trigger
  Counter2/1 -> OR1/1
  Multiply/1 -> Edge Detector Rise/Fall/1(In), OR1/2, Sample and Hold/1, Scope/1
  Edge Detector Rise/Fall/1(Out) -> Counter2/2
  Counter1/1 -> Compare To Constant/1
  Input/1 -> Rate Transition/1
  Rate Transition/1 -> Multiply/2, AND/1, Edge Detector1/1
  NOT/1 -> Edge Detector2/1
  Edge Detector2/1 -> AND/2
  AND/1 -> OR/2
  OR/1 -> Counter1/2
  Edge Detector1/1 -> OR/1
  Delay/1 -> NOT/1
  Compare To Constant/1 -> Multiply/1

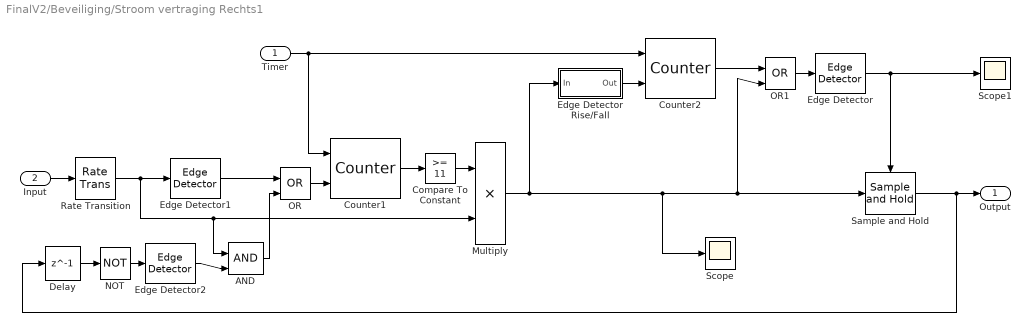
== system FinalV2/Beveiliging/Stroom vertraging Rechts1 ==
  Timer : Inport
  Input : Inport  Port=2
  AND : Logic  IconShape=distinctive  AllPortsSameDT=off  OutDataTypeStr=boolean
  Compare To Constant : simulink/Logic and Bit Operations/Compare To Constant  relop=>=  const=11  OutDataTypeStr=boolean
  Counter1 : dspswit3/Counter  Direction=Up  CountEvent=Rising edge  CounterSize=32 bits  MaxCount=20  InitialCount=0  Output=Count  HitValue=20  ResetInput=on  SamplesPerFrame=1  Ts=1  CntDtype=double  HitDtype=Logical
  Counter2 : dspswit3/Counter  Direction=Up  CountEvent=Rising edge  CounterSize=User defined  MaxCount=201  InitialCount=0  Output=Hit  HitValue=201  ResetInput=on  SamplesPerFrame=1  Ts=1  CntDtype=double  HitDtype=Logical
  Delay : Delay  DelayLength=1
  Edge Detector : dspswit3/Edge Detector  InputProcessing=Columns as channels (frame based)
      settings: SourceProductName=DSP System Toolbox  SourceProductBaseCode=DS
  Edge Detector1 : dspswit3/Edge Detector  InputProcessing=Columns as channels (frame based)
      settings: SourceProductName=DSP System Toolbox  SourceProductBaseCode=DS
  Edge Detector2 : dspswit3/Edge Detector  InputProcessing=Columns as channels (frame based)
      settings: SourceProductName=DSP System Toolbox  SourceProductBaseCode=DS
  Edge Detector Rise/Fall : Subsystem
  Multiply : Product
  NOT : Logic  Operator=NOT  IconShape=distinctive  AllPortsSameDT=off  OutDataTypeStr=boolean
  OR : Logic  Operator=OR  IconShape=distinctive  AllPortsSameDT=off  OutDataTypeStr=boolean
  OR1 : Logic  Operator=OR  IconShape=distinctive  AllPortsSameDT=off  OutDataTypeStr=boolean
  Rate Transition : RateTransition  OutPortSampleTime=1/1000
  Sample and Hold : dspsigops/Sample and Hold  trig=Rising edge  initCond=0  latchinput=off
  Scope : Scope
  Scope1 : Scope
  Output : Outport
  wires:
  Timer/1 -> Counter2/1, Counter1/1
  Sample and Hold/1 -> Output/1, Delay/1
  OR1/1 -> Edge Detector/1
  Edge Detector/1 -> Scope1/1, Sample and Hold/Trigger
  Counter2/1 -> OR1/1
  Multiply/1 -> Edge Detector Rise/Fall/1(In), OR1/2, Sample and Hold/1, Scope/1
  Edge Detector Rise/Fall/1(Out) -> Counter2/2
  Counter1/1 -> Compare To Constant/1
  Input/1 -> Rate Transition/1
  Rate Transition/1 -> Multiply/2, AND/1, Edge Detector1/1
  NOT/1 -> Edge Detector2/1
  Edge Detector2/1 -> AND/2
  AND/1 -> OR/2
  OR/1 -> Counter1/2
  Edge Detector1/1 -> OR/1
  Delay/1 -> NOT/1
  Compare To Constant/1 -> Multiply/1

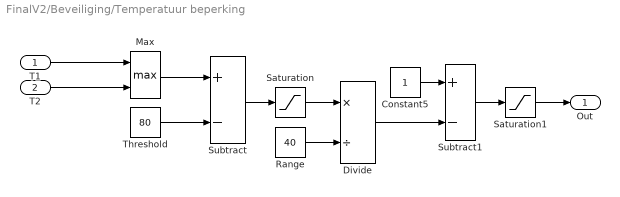
== system FinalV2/Beveiliging/Temperatuur beperking ==
  T1 : Inport
  T2 : Inport  Port=2
  Constant5 : Constant
  Divide : Product  Inputs=*/
  Max : MinMax  Function=max  Inputs=2
  Range : Constant  Value=40
  Saturation : Saturate  UpperLimit=inf  LowerLimit=0
  Saturation1 : Saturate  UpperLimit=1  LowerLimit=0
  Subtract : Sum  Inputs=+-
  Subtract1 : Sum  Inputs=+-
  Threshold : Constant  Value=80
  Out : Outport
  wires:
  Subtract/1 -> Saturation/1
  Divide/1 -> Subtract1/2
  Constant5/1 -> Subtract1/1
  Threshold/1 -> Subtract/2
  Max/1 -> Subtract/1
  T2/1 -> Max/2
  Range/1 -> Divide/2
  Saturation/1 -> Divide/1
  Subtract1/1 -> Saturation1/1
  T1/1 -> Max/1
  Saturation1/1 -> Out/1

== system FinalV2/Beveiliging/Temperatuur vertraging Links ==
  Timer : Inport
  Input : Inport  Port=2
  Counter2 : dspswit3/Counter  Direction=Up  CountEvent=Rising edge  CounterSize=User defined  MaxCount=300  InitialCount=0  Output=Hit  HitValue=300  ResetInput=on  SamplesPerFrame=1  Ts=1  CntDtype=double  HitDtype=Logical
  Edge Detector : dspswit3/Edge Detector  InputProcessing=Columns as channels (frame based)
      settings: SourceProductName=DSP System Toolbox  SourceProductBaseCode=DS
  Edge Detector Rise/Fall : Subsystem
  OR1 : Logic  Operator=OR  IconShape=distinctive  AllPortsSameDT=off  OutDataTypeStr=boolean
  Sample and Hold : dspsigops/Sample and Hold  trig=Rising edge  initCond=0  latchinput=off
  Scope : Scope
  Scope1 : Scope
  Output : Outport
  wires:
  Timer/1 -> Counter2/1
  Sample and Hold/1 -> Output/1
  OR1/1 -> Edge Detector/1
  Edge Detector/1 -> Scope1/1, Sample and Hold/Trigger
  Counter2/1 -> OR1/1
  Input/1 -> Scope/1, OR1/2, Sample and Hold/1, Edge Detector Rise/Fall/1(In)
  Edge Detector Rise/Fall/1(Out) -> Counter2/2

== system FinalV2/Beveiliging/Temperatuur vertraging Rechts  ==
  Timer : Inport
  Input : Inport  Port=2
  Counter2 : dspswit3/Counter  Direction=Up  CountEvent=Rising edge  CounterSize=User defined  MaxCount=300  InitialCount=0  Output=Hit  HitValue=300  ResetInput=on  SamplesPerFrame=1  Ts=1  CntDtype=double  HitDtype=Logical
  Edge Detector : dspswit3/Edge Detector  InputProcessing=Columns as channels (frame based)
      settings: SourceProductName=DSP System Toolbox  SourceProductBaseCode=DS
  Edge Detector Rise/Fall : Subsystem
  OR1 : Logic  Operator=OR  IconShape=distinctive  AllPortsSameDT=off  OutDataTypeStr=boolean
  Sample and Hold : dspsigops/Sample and Hold  trig=Rising edge  initCond=0  latchinput=off
  Scope : Scope
  Scope1 : Scope
  Output : Outport
  wires:
  Timer/1 -> Counter2/1
  Sample and Hold/1 -> Output/1
  OR1/1 -> Edge Detector/1
  Edge Detector/1 -> Scope1/1, Sample and Hold/Trigger
  Counter2/1 -> OR1/1
  Input/1 -> Scope/1, OR1/2, Sample and Hold/1, Edge Detector Rise/Fall/1(In)
  Edge Detector Rise/Fall/1(Out) -> Counter2/2

== system FinalV2/Stuurhoek Converter/Output > 100% ==
  L_In : Inport
  R_In : Inport  Port=2
  Compare To Constant : simulink/Logic and Bit Operations/Compare To Constant  relop=>  const=1  OutDataTypeStr=boolean
  Compare To Constant1 : simulink/Logic and Bit Operations/Compare To Constant  relop=>  const=1  OutDataTypeStr=boolean
  Divide4 : Product  Inputs=**
  Divide5 : Product  Inputs=**
  Subtract : Sum  Inputs=+-
  Subtract1 : Sum  Inputs=-+
  L_Out : Outport
  R_Out : Outport  Port=2
  wires:
  Compare To Constant1/1 -> Subtract1/1, Divide4/1
  Compare To Constant/1 -> Subtract/2, Divide5/2
  Subtract1/1 -> Divide4/2
  Subtract/1 -> Divide5/1
  L_In/1 -> Subtract/1, Compare To Constant/1
  Divide5/1 -> R_Out/1
  R_In/1 -> Subtract1/2, Compare To Constant1/1
  Divide4/1 -> L_Out/1

== system FinalV2/Beveiliging/Stroom vertraging Rechts/Edge Detector Rise//Fall ==
  In : Inport
  Edge Detector1 : dspswit3/Edge Detector  InputProcessing=Columns as channels (frame based)
      settings: SourceProductName=DSP System Toolbox  SourceProductBaseCode=DS
  Edge Detector2 : dspswit3/Edge Detector  InputProcessing=Columns as channels (frame based)
      settings: SourceProductName=DSP System Toolbox  SourceProductBaseCode=DS
  NOT : Logic  Operator=NOT  IconShape=distinctive  AllPortsSameDT=off  OutDataTypeStr=boolean
  OR : Logic  Operator=OR  IconShape=distinctive  AllPortsSameDT=off  OutDataTypeStr=boolean
  Out : Outport
  wires:
  In/1 -> NOT/1, Edge Detector1/1
  NOT/1 -> Edge Detector2/1
  Edge Detector1/1 -> OR/1
  OR/1 -> Out/1
  Edge Detector2/1 -> OR/2

== system FinalV2/Beveiliging/Stroom vertraging Rechts1/Edge Detector Rise//Fall ==
  In : Inport
  Edge Detector1 : dspswit3/Edge Detector  InputProcessing=Columns as channels (frame based)
      settings: SourceProductName=DSP System Toolbox  SourceProductBaseCode=DS
  Edge Detector2 : dspswit3/Edge Detector  InputProcessing=Columns as channels (frame based)
      settings: SourceProductName=DSP System Toolbox  SourceProductBaseCode=DS
  NOT : Logic  Operator=NOT  IconShape=distinctive  AllPortsSameDT=off  OutDataTypeStr=boolean
  OR : Logic  Operator=OR  IconShape=distinctive  AllPortsSameDT=off  OutDataTypeStr=boolean
  Out : Outport
  wires:
  In/1 -> NOT/1, Edge Detector1/1
  NOT/1 -> Edge Detector2/1
  Edge Detector1/1 -> OR/1
  OR/1 -> Out/1
  Edge Detector2/1 -> OR/2

== system FinalV2/Beveiliging/Temperatuur vertraging Links/Edge Detector Rise//Fall ==
  In : Inport
  Edge Detector1 : dspswit3/Edge Detector  InputProcessing=Columns as channels (frame based)
      settings: SourceProductName=DSP System Toolbox  SourceProductBaseCode=DS
  Edge Detector2 : dspswit3/Edge Detector  InputProcessing=Columns as channels (frame based)
      settings: SourceProductName=DSP System Toolbox  SourceProductBaseCode=DS
  NOT : Logic  Operator=NOT  IconShape=distinctive  AllPortsSameDT=off  OutDataTypeStr=boolean
  OR : Logic  Operator=OR  IconShape=distinctive  AllPortsSameDT=off  OutDataTypeStr=boolean
  Out : Outport
  wires:
  In/1 -> NOT/1, Edge Detector1/1
  NOT/1 -> Edge Detector2/1
  Edge Detector1/1 -> OR/1
  OR/1 -> Out/1
  Edge Detector2/1 -> OR/2

== system FinalV2/Beveiliging/Temperatuur vertraging Rechts /Edge Detector Rise//Fall ==
  In : Inport
  Edge Detector1 : dspswit3/Edge Detector  InputProcessing=Columns as channels (frame based)
      settings: SourceProductName=DSP System Toolbox  SourceProductBaseCode=DS
  Edge Detector2 : dspswit3/Edge Detector  InputProcessing=Columns as channels (frame based)
      settings: SourceProductName=DSP System Toolbox  SourceProductBaseCode=DS
  NOT : Logic  Operator=NOT  IconShape=distinctive  AllPortsSameDT=off  OutDataTypeStr=boolean
  OR : Logic  Operator=OR  IconShape=distinctive  AllPortsSameDT=off  OutDataTypeStr=boolean
  Out : Outport
  wires:
  In/1 -> NOT/1, Edge Detector1/1
  NOT/1 -> Edge Detector2/1
  Edge Detector1/1 -> OR/1
  OR/1 -> Out/1
  Edge Detector2/1 -> OR/2

== matlab function FinalV2/Snelheidsmeter Rechts/Periode meting ==
  data: speedPulse input; pulses output; speedPulseBuf data_store_memory; pulseCount data_store_memory; period input; i data_store_memory; fs input; j data_store_memory; reset input
function pulses = fcn(speedPulse,period, fs, reset)

global pulseCount;
global speedPulseBuf;
global i;
global j;

if reset == 1
    speedPulseBuf = uint8(zeros(size(speedPulseBuf)));
end

bufTime = period*fs + 1;

if i > bufTime
    i = uint32(1);
end

if j > bufTime
    j = uint32(1);
end

speedPulseBuf(i) = speedPulse;
pulseCount = pulseCount + uint32(speedPulse);
pulseCount = pulseCount - uint32(speedPulseBuf(j));

i = i + 1;
j = j + 1;

pulses = pulseCount;
